simulink model "pry_grasp_source"  (R2018b)
settings: Solver=FixedStepDiscrete  StartTime=0.0  StopTime=Inf  FixedStep=0.001  RelTol=1e-3
PostLoadFcn:
  | , if any(exist('dsrtsu_mdlpostloadfcn', 'file') ~= 0), dsrtsu_mdlpostloadfcn('Execute', bdroot); end,
undefined symbols (not defined in the file): b, Coulomb_friction, parallel_grasp, q1ini, q2ini, theta1, theta2, theta5, theta6, viscous_friction
libraries: simulink x26
(part 3 of 3)

== system pry_grasp_source/phase700/Enabled Subsystem7/Subsystem ==
  note: 关节6弹簧特性
  note: 关节5弹簧特性
  initial_angle : Inport
  end_angle : Inport  Port=2
  end_time : Inport  Port=3
  time : Inport  Port=4
  angular_vel : Inport  Port=5
  current_angle : Inport  Port=6
  Enable : EnablePort
  Demux : Demux  Outputs=8
  Demux1 : Demux  Outputs=8
  MATLAB Function : MATLAB Function  TreatAsAtomicUnit=on
  Mux : Mux  Inputs=8
  P5 : Subsystem
  P6 : Subsystem
  PID1 : Subsystem
  PID2 : Subsystem
  PID3 : Subsystem
  PID4 : Subsystem
  PID7 : Subsystem
  PID8 : Subsystem
  Sum2 : Sum  Inputs=|+-
  angle2 down1 : Constant  Value=2
  angle2 down2 : Constant  Value=2
  torque_out : Outport  OutputWhenDisabled=reset  InitialOutput=[0 0 0 0 0 0 0 0]
  wires:
  initial_angle/1 -> MATLAB Function/1(initial_q)
  end_angle/1 -> MATLAB Function/2(end_q)
  time/1 -> MATLAB Function/4(time)
  end_time/1 -> MATLAB Function/3(end_time)
  angular_vel/1 -> Demux1/1
  MATLAB Function/1(angle_ref_out) -> Sum2/1
  Sum2/1 -> Demux/1
  current_angle/1 -> Sum2/2
  Mux/1 -> torque_out/1
  Demux/1 -> PID1/1(angle_error)
  Demux1/1 -> PID1/2(angular_vel)
  PID1/1(torque) -> Mux/1
  Demux/3 -> PID3/1(angle_error)
  Demux/4 -> PID4/1(angle_error)
  PID3/1(torque) -> Mux/3
  PID4/1(torque) -> Mux/4
  Demux1/3 -> PID3/2(angular_vel)
  Demux1/4 -> PID4/2(angular_vel)
  Demux/7 -> PID7/1(angle_error)
  Demux/8 -> PID8/1(angle_error)
  PID7/1(torque) -> Mux/7
  PID8/1(torque) -> Mux/8
  Demux1/7 -> PID7/2(angular_vel)
  Demux1/8 -> PID8/2(angular_vel)
  PID2/1(torque) -> Mux/2
  angle2 down1/1 -> P6/1(angle_error)
  P6/1(torque6) -> Mux/6
  P5/1(torque6) -> Mux/5
  Demux/2 -> PID2/1(angle_error)
  Demux1/2 -> PID2/2(angular_vel)
  angle2 down2/1 -> P5/1(angle_error)

== system pry_grasp_source/phase700/Enabled Subsystem7/Triggered Subsystem ==
  angle_In1 : Inport
  angle_ref_In2 : Inport  Port=2
  end_time_In3 : Inport  Port=3
  Trigger : TriggerPort  VariantControl=Variant
  angle_Out1 : Outport  InitialOutput=0
  angle_ref_Out2 : Outport  Port=2  InitialOutput=0
  end_time_Out3 : Outport  Port=3  InitialOutput=0
  wires:
  angle_In1/1 -> angle_Out1/1
  angle_ref_In2/1 -> angle_ref_Out2/1
  end_time_In3/1 -> end_time_Out3/1

== system pry_grasp_source/phase700/Subsystem1/Triggered Subsystem3 ==
  Trigger : TriggerPort  VariantControl=(inherit)
  Constant : Constant  Value=[0 1]
  Data Store Read : DataStoreRead  Priority=3  DataStoreName=phase_num
  Data Store Write : DataStoreWrite  DataStoreName=phase_num
  Sum : Sum  Inputs=|++
  wires:
  Data Store Read/1 -> Sum/1
  Sum/1 -> Data Store Write/1
  Constant/1 -> Sum/2

== system pry_grasp_source/phase90/Enabled Subsystem4/Subsystem1 ==
  note: 使关节5平滑转到相应角度
  note: 使关节2维持相应角度
  note: 关节6弹簧特性
  note: 关节2维持角度
  initial_angle5 : Inport
  end_angle5 : Inport  Port=2
  end_time : Inport  Port=3
  time : Inport  Port=4
  angular5_vel : Inport  Port=5
  current_angle5 : Inport  Port=6
  "angle2 " : Inport  Port=7
  angle1 : Inport  Port=8
  Enable : EnablePort
  Fx_1 : Constant
  Fy_1 : Constant  Value=0.1
  MATLAB Function : MATLAB Function  TreatAsAtomicUnit=on
  MATLAB Function1 : MATLAB Function  TreatAsAtomicUnit=on
  Mux : Mux  Inputs=8
  P6 : Subsystem
  PID5 : Subsystem
  Sum2 : Sum  Inputs=|+-
  angle6 down : Constant  Value=-2
  other tau : Constant  Value=0
  phi_value : Constant  Value=16
  torque : Outport
  wires:
  end_time/1 -> MATLAB Function/3(end_time)
  Sum2/1 -> PID5/1(angle_error)
  initial_angle5/1 -> MATLAB Function/1(initial_q)
  time/1 -> MATLAB Function/4(time)
  current_angle5/1 -> Sum2/2
  angular5_vel/1 -> PID5/2(angular_vel)
  MATLAB Function/1(angle_ref_out) -> Sum2/1
  end_angle5/1 -> MATLAB Function/2(end_q)
  angle6 down/1 -> P6/1(angle_error)
  phi_value/1 -> MATLAB Function1/1(phi_value)
  Mux/1 -> torque/1
  other tau/1 -> Mux/8, Mux/7, Mux/4, Mux/3
  PID5/1(torque) -> Mux/5
  P6/1(torque1) -> Mux/6
  Fx_1/1 -> MATLAB Function1/2(Fx_1)
  Fy_1/1 -> MATLAB Function1/3(Fy_1)
  "angle2 "/1 -> MATLAB Function1/5(theta2_value)
  angle1/1 -> MATLAB Function1/4(theta1_value)
  MATLAB Function1/1(tau1) -> Mux/1
  MATLAB Function1/2(tau2) -> Mux/2

== system pry_grasp_source/phase90/Enabled Subsystem4/Triggered Subsystem ==
  angle5_In : Inport
  angle5_ref : Inport  Port=2
  end_time : Inport  Port=3
  Trigger : TriggerPort  VariantControl=Variant
  angle5_Out : Outport  InitialOutput=0
  angle5_ref_Out : Outport  Port=2  InitialOutput=0
  end_time_Out : Outport  Port=3  InitialOutput=0
  wires:
  angle5_In/1 -> angle5_Out/1
  angle5_ref/1 -> angle5_ref_Out/1
  end_time/1 -> end_time_Out/1

== system pry_grasp_source/prying motion/Enabled Subsystem4/Subsystem1 ==
  pry force : Inport
  "angle2 " : Inport  Port=2
  angle1 : Inport  Port=3
  angle6 : Inport  Port=4
  angle5 : Inport  Port=5
  Enable : EnablePort
  Fy_1_finger1 : Constant  Value=0.1
  Fy_1_finger2 : Constant  Value=0.1
  MATLAB Function1 : MATLAB Function  TreatAsAtomicUnit=on
  MATLAB Function2 : MATLAB Function  TreatAsAtomicUnit=on
  Mux : Mux
  offset : Gain  Gain=0.3
  torque : Outport
  wires:
  Mux/1 -> torque/1
  MATLAB Function1/2(tau2) -> Mux/2
  angle1/1 -> MATLAB Function1/3(theta1_value)
  MATLAB Function1/1(tau1) -> Mux/1
  Fy_1_finger1/1 -> MATLAB Function1/2(Fy_1)
  "angle2 "/1 -> MATLAB Function1/4(theta2_value)
  pry force/1 -> offset/1, MATLAB Function1/1(Fx_1)
  angle6/1 -> MATLAB Function2/4(theta6)
  Fy_1_finger2/1 -> MATLAB Function2/2(Fy_1)
  angle5/1 -> MATLAB Function2/3(theta5)
  offset/1 -> MATLAB Function2/1(Fx_1)
  MATLAB Function2/1(tau5) -> Mux/3
  MATLAB Function2/2(tau6) -> Mux/4

== system pry_grasp_source/pusher drops to detect the table surface/friction_compensation model/PID1 ==
  angle_error : Inport
  angular_vel : Inport  Port=2
  Data Store Read : DataStoreRead  DataStoreName=gain1
  Kd : Gain  Gain=0.0005
  Kp : Gain  Gain=0.15
  Product : Product
  Sum1 : Sum  Inputs=|+-
  torque : Outport
  wires:
  Kd/1 -> Sum1/2
  Sum1/1 -> Product/1
  Product/1 -> torque/1
  Kp/1 -> Sum1/1
  angle_error/1 -> Kp/1
  angular_vel/1 -> Kd/1
  Data Store Read/1 -> Product/2

== system pry_grasp_source/pusher drops to detect the table surface/friction_compensation model/PID2 ==
  angle_error : Inport
  angular_vel : Inport  Port=2
  Data Store Read : DataStoreRead  DataStoreName=gain2
  Kd : Gain  Gain=0.0005
  Kp : Gain  Gain=0.15
  Product : Product
  Sum1 : Sum  Inputs=|+-
  torque : Outport
  wires:
  Kd/1 -> Sum1/2
  Sum1/1 -> Product/1
  Product/1 -> torque/1
  Kp/1 -> Sum1/1
  angle_error/1 -> Kp/1
  angular_vel/1 -> Kd/1
  Data Store Read/1 -> Product/2

== system pry_grasp_source/pusher drops to detect the table surface/friction_compensation model/PID6 ==
  angle_error : Inport
  angular_vel : Inport  Port=2
  Data Store Read : DataStoreRead  DataStoreName=gain6
  Kd : Gain  Gain=0.0005
  Kp : Gain  Gain=0.15
  Product : Product
  Sum1 : Sum  Inputs=|+-
  torque : Outport
  wires:
  Kd/1 -> Sum1/2
  Sum1/1 -> Product/1
  Product/1 -> torque/1
  Kp/1 -> Sum1/1
  angle_error/1 -> Kp/1
  angular_vel/1 -> Kd/1
  Data Store Read/1 -> Product/2

== system pry_grasp_source/pusher drops to detect the table surface/friction_compensation model/joint5 torque compensation1 ==
  angular_velocity : Inport
  C5 : Constant  Value=Coulomb_friction  SampleTime=-1
  D5 : Constant  Value=viscous_friction  SampleTime=-1
  Stribeck_friction_model : MATLAB Function  TreatAsAtomicUnit=on
  torque_out : Outport  OutputWhenDisabled=reset  InitialOutput=0
  wires:
  angular_velocity/1 -> Stribeck_friction_model/3(angular_vel)
  C5/1 -> Stribeck_friction_model/1(C)
  D5/1 -> Stribeck_friction_model/2(D)
  Stribeck_friction_model/1(torque_out) -> torque_out/1

== system pry_grasp_source/pusher pushes object/Subsystem1/Triggered Subsystem3 ==
  Trigger : TriggerPort  VariantControl=(inherit)
  Constant : Constant  Value=[0 1]
  Data Store Read : DataStoreRead  Priority=3  DataStoreName=phase_num
  Data Store Write : DataStoreWrite  DataStoreName=phase_num
  Sum : Sum  Inputs=|++
  wires:
  Data Store Read/1 -> Sum/1
  Sum/1 -> Data Store Write/1
  Constant/1 -> Sum/2

== system pry_grasp_source/return to initial angle/Enabled Subsystem7/Subsystem ==
  initial_angle : Inport
  end_angle : Inport  Port=2
  end_time : Inport  Port=3
  time : Inport  Port=4
  angular_vel : Inport  Port=5
  current_angle : Inport  Port=6
  Enable : EnablePort
  Demux : Demux  Outputs=1
  Demux1 : Demux  Outputs=1
  MATLAB Function : MATLAB Function  TreatAsAtomicUnit=on
  Mux : Mux
  PID2 : Subsystem
  Sum2 : Sum  Inputs=|+-
  torque_out : Outport  OutputWhenDisabled=reset  InitialOutput=[0 0 0 0 0 0 0 0]
  wires:
  initial_angle/1 -> MATLAB Function/1(initial_q)
  end_angle/1 -> MATLAB Function/2(end_q)
  time/1 -> MATLAB Function/4(time)
  end_time/1 -> MATLAB Function/3(end_time)
  angular_vel/1 -> Demux1/1
  MATLAB Function/1(angle_ref_out) -> Sum2/1
  Sum2/1 -> Demux/1
  current_angle/1 -> Sum2/2
  Mux/1 -> torque_out/1
  Demux/1 -> PID2/1(angle_error)
  PID2/1(torque) -> Mux/2
  Demux1/1 -> PID2/2(angular_vel)

== system pry_grasp_source/return to initial angle/Enabled Subsystem7/Triggered Subsystem ==
  angle_In1 : Inport
  angle_ref_In2 : Inport  Port=2
  end_time_In3 : Inport  Port=3
  Trigger : TriggerPort  VariantControl=Variant
  angle_Out1 : Outport  InitialOutput=0
  angle_ref_Out2 : Outport  Port=2  InitialOutput=0
  end_time_Out3 : Outport  Port=3  InitialOutput=0
  wires:
  angle_In1/1 -> angle_Out1/1
  angle_ref_In2/1 -> angle_ref_Out2/1
  end_time_In3/1 -> end_time_Out3/1

== system pry_grasp_source/return to initial position/Enabled Subsystem7/Subsystem ==
  initial_angle : Inport
  end_angle : Inport  Port=2
  end_time : Inport  Port=3
  time : Inport  Port=4
  angular_vel : Inport  Port=5
  current_angle : Inport  Port=6
  Enable : EnablePort
  Demux : Demux  Outputs=1
  MATLAB Function : MATLAB Function  TreatAsAtomicUnit=on
  Mux : Mux
  PID1 : Subsystem
  Sum2 : Sum  Inputs=|+-
  tau1 : Gain
  tau_out : Outport
  wires:
  initial_angle/1 -> MATLAB Function/1(initial_q)
  end_angle/1 -> MATLAB Function/2(end_q)
  time/1 -> MATLAB Function/4(time)
  end_time/1 -> MATLAB Function/3(end_time)
  MATLAB Function/1(angle_ref_out) -> Sum2/1
  Sum2/1 -> Demux/1
  current_angle/1 -> Sum2/2
  Mux/1 -> tau_out/1
  Demux/1 -> PID1/1(angle_error)
  angular_vel/1 -> PID1/2(angular_vel)
  PID1/1(torque) -> tau1/1, Mux/1

== system pry_grasp_source/return to initial position/Enabled Subsystem7/Triggered Subsystem ==
  angle_In1 : Inport
  angle_ref_In2 : Inport  Port=2
  end_time_In3 : Inport  Port=3
  Trigger : TriggerPort  VariantControl=Variant
  angle_Out1 : Outport  InitialOutput=0
  angle_ref_Out2 : Outport  Port=2  InitialOutput=0
  end_time_Out3 : Outport  Port=3  InitialOutput=0
  wires:
  angle_In1/1 -> angle_Out1/1
  angle_ref_In2/1 -> angle_ref_Out2/1
  end_time_In3/1 -> end_time_Out3/1

== system pry_grasp_source/tentatively push/Enabled Subsystem1/Subsystem1 ==
  note: 使关节5平滑转到相应角度
  note: desired y
  initial angle : Inport
  end_angle : Inport  Port=2
  end_time : Inport  Port=3
  time : Inport  Port=4
  current angle : Inport  Port=5
  angular_vel : Inport  Port=6
  phase time : Inport  Port=7
  Enable : EnablePort
  Constant2 : Constant  Value=0
  Demux : Demux  Outputs=8
  Demux1 : Demux  Outputs=2
  Gain : Gain  Gain=b
  MATLAB Function : MATLAB Function  TreatAsAtomicUnit=on
  MATLAB Function3 : MATLAB Function  TreatAsAtomicUnit=on
  MATLAB Function4 : MATLAB Function  TreatAsAtomicUnit=on
  Mux : Mux
  Mux{1..4} (4 alike) : Mux  Inputs=2
  PID1 : Subsystem
  PID2 : Subsystem
  Sum : Sum  Inputs=|+-
  Sum1 : Sum  Inputs=|+-
  Sum2 : Sum  Inputs=|+-
  Sum3 : Sum  Inputs=|++
  Sum4 : Sum  Inputs=|++
  measured Fx : Constant  Value=0
  measured Fy : Constant  Value=0.1
  torque : Outport
  wires:
  end_time/1 -> MATLAB Function/3(end_time)
  initial angle/1 -> MATLAB Function/1(initial_q)
  time/1 -> MATLAB Function/4(time)
  current angle/1 -> Sum2/2
  MATLAB Function/1(angle_ref_out) -> Sum2/1
  end_angle/1 -> MATLAB Function/2(end_q)
  Mux/1 -> torque/1
  PID1/1(torque) -> Mux/1
  PID2/1(torque) -> Mux/2
  Sum2/1 -> Demux/1
  Demux/1 -> PID1/1(angle_error)
  Demux/2 -> PID2/1(angle_error)
  angular_vel/1 -> Demux1/1
  Demux1/1 -> PID1/2(angular_vel)
  Demux1/2 -> PID2/2(angular_vel)
  Mux1/1 -> Sum/1
  measured Fy/1 -> Mux2/2
  Mux2/1 -> Sum/2
  MATLAB Function3/2(tau6f) -> Sum4/2
  MATLAB Function4/1(tau5s) -> Sum3/1
  Mux3/1 -> Sum1/1
  Sum/1 -> MATLAB Function3/1(F_e)
  measured Fx/1 -> Mux2/1
  [P_x] -> Mux4/1
  Sum1/1 -> MATLAB Function4/1(P_e)
  [P_y] -> Mux4/2
  Gain/1 -> Mux3/1
  MATLAB Function3/1(tau5f) -> Sum3/2
  Constant2/1 -> Mux3/2
  MATLAB Function4/2(tau6s) -> Sum4/1
  [F_yd] -> Mux1/2
  phase time/1 -> Gain/1
  Sum4/1 -> Mux/4
  [F_xd] -> Mux1/1
  Mux4/1 -> Sum1/2
  Sum3/1 -> Mux/3

== system pry_grasp_source/tentatively push/Enabled Subsystem1/Triggered Subsystem ==
  angle_In : Inport
  angle_ref : Inport  Port=2
  end_time : Inport  Port=3
  Trigger : TriggerPort  VariantControl=Variant
  angle_Out : Outport  InitialOutput=0
  angle_ref_Out : Outport  Port=2  InitialOutput=0
  end_time_Out : Outport  Port=3  InitialOutput=0
  wires:
  angle_In/1 -> angle_Out/1
  angle_ref/1 -> angle_ref_Out/1
  end_time/1 -> end_time_Out/1

== system pry_grasp_source/phase1/Enabled Subsystem7/Subsystem/PID1 ==
  angle_error : Inport
  angular_vel : Inport  Port=2
  Data Store Read : DataStoreRead  DataStoreName=gain1
  Kd : Gain  Gain=0.0005
  Kp : Gain  Gain=0.15
  Product : Product
  Sum1 : Sum  Inputs=|+-
  torque : Outport
  wires:
  Kd/1 -> Sum1/2
  Sum1/1 -> Product/1
  Product/1 -> torque/1
  Kp/1 -> Sum1/1
  angle_error/1 -> Kp/1
  angular_vel/1 -> Kd/1
  Data Store Read/1 -> Product/2

== system pry_grasp_source/phase1/Enabled Subsystem7/Subsystem/PID2 ==
  angle_error : Inport
  angular_vel : Inport  Port=2
  Data Store Read : DataStoreRead  DataStoreName=gain2
  Kd2 : Gain  Gain=0.0002
  Kp2 : Gain  Gain=0.08
  Product : Product
  Sum1 : Sum  Inputs=|+-
  torque : Outport
  wires:
  Kp2/1 -> Sum1/1
  angular_vel/1 -> Kd2/1
  Product/1 -> torque/1
  Kd2/1 -> Sum1/2
  angle_error/1 -> Kp2/1
  Data Store Read/1 -> Product/2
  Sum1/1 -> Product/1

== system pry_grasp_source/phase1/Enabled Subsystem7/Subsystem/PID3 ==
  angle_error : Inport
  angular_vel : Inport  Port=2
  Kd : Gain  Gain=0.0005
  Kp : Gain  Gain=0.15
  Sum1 : Sum  Inputs=|+-
  gain : Gain  Gain=0.5
  torque : Outport
  wires:
  Kd/1 -> Sum1/2
  Sum1/1 -> gain/1
  gain/1 -> torque/1
  Kp/1 -> Sum1/1
  angle_error/1 -> Kp/1
  angular_vel/1 -> Kd/1

== system pry_grasp_source/phase1/Enabled Subsystem7/Subsystem/PID4 ==
  angle_error : Inport
  angular_vel : Inport  Port=2
  Kd2 : Gain  Gain=0.0002
  Kp2 : Gain  Gain=0.08
  Sum1 : Sum  Inputs=|+-
  gain : Gain  Gain=0.5
  torque : Outport
  wires:
  Kp2/1 -> Sum1/1
  angular_vel/1 -> Kd2/1
  Sum1/1 -> gain/1
  gain/1 -> torque/1
  Kd2/1 -> Sum1/2
  angle_error/1 -> Kp2/1

== system pry_grasp_source/phase1/Enabled Subsystem7/Subsystem/PID5 ==
  angle_error : Inport
  angular_vel : Inport  Port=2
  Data Store Read : DataStoreRead  DataStoreName=gain5
  Kd : Gain  Gain=0.0005
  Kp : Gain  Gain=0.15
  Product : Product
  Sum1 : Sum  Inputs=|+-
  torque : Outport
  wires:
  Kd/1 -> Sum1/2
  Kp/1 -> Sum1/1
  angle_error/1 -> Kp/1
  angular_vel/1 -> Kd/1
  Data Store Read/1 -> Product/2
  Sum1/1 -> Product/1
  Product/1 -> torque/1

== system pry_grasp_source/phase1/Enabled Subsystem7/Subsystem/PID6 ==
  angle_error : Inport
  angular_vel : Inport  Port=2
  Data Store Read : DataStoreRead  DataStoreName=gain6
  Kd2 : Gain  Gain=0.0002
  Kp2 : Gain  Gain=0.08
  Product : Product
  Sum1 : Sum  Inputs=|+-
  torque : Outport
  wires:
  Kp2/1 -> Sum1/1
  angular_vel/1 -> Kd2/1
  Sum1/1 -> Product/1
  Product/1 -> torque/1
  Kd2/1 -> Sum1/2
  angle_error/1 -> Kp2/1
  Data Store Read/1 -> Product/2

== system pry_grasp_source/phase1/Enabled Subsystem7/Subsystem/PID7 ==
  angle_error : Inport
  angular_vel : Inport  Port=2
  Kd : Gain  Gain=0.0005
  Kp : Gain  Gain=0.15
  Sum1 : Sum  Inputs=|+-
  gain : Gain  Gain=0.5
  torque : Outport
  wires:
  Kd/1 -> Sum1/2
  Sum1/1 -> gain/1
  gain/1 -> torque/1
  Kp/1 -> Sum1/1
  angle_error/1 -> Kp/1
  angular_vel/1 -> Kd/1

== system pry_grasp_source/phase1/Enabled Subsystem7/Subsystem/PID8 ==
  angle_error : Inport
  angular_vel : Inport  Port=2
  Kd : Gain  Gain=0.0005
  Kp : Gain  Gain=0.15
  Sum1 : Sum  Inputs=|+-
  gain : Gain  Gain=0.5
  torque : Outport
  wires:
  Kd/1 -> Sum1/2
  Sum1/1 -> gain/1
  gain/1 -> torque/1
  Kp/1 -> Sum1/1
  angle_error/1 -> Kp/1
  angular_vel/1 -> Kd/1

== system pry_grasp_source/phase1-1/Enabled Subsystem7/Subsystem/PID1 ==
  angle_error : Inport
  angular_vel : Inport  Port=2
  Data Store Read : DataStoreRead  DataStoreName=gain1
  Kd : Gain  Gain=0.0005
  Kp : Gain  Gain=0.15
  Product : Product
  Sum1 : Sum  Inputs=|+-
  torque : Outport
  wires:
  Kd/1 -> Sum1/2
  Sum1/1 -> Product/1
  Product/1 -> torque/1
  Kp/1 -> Sum1/1
  angle_error/1 -> Kp/1
  angular_vel/1 -> Kd/1
  Data Store Read/1 -> Product/2

== system pry_grasp_source/phase1-1/Enabled Subsystem7/Subsystem/PID2 ==
  angle_error : Inport
  angular_vel : Inport  Port=2
  Data Store Read : DataStoreRead  DataStoreName=gain2
  Kd2 : Gain  Gain=0.0002
  Kp2 : Gain  Gain=0.08
  Product : Product
  Sum1 : Sum  Inputs=|+-
  torque : Outport
  wires:
  Kp2/1 -> Sum1/1
  angular_vel/1 -> Kd2/1
  Product/1 -> torque/1
  Kd2/1 -> Sum1/2
  angle_error/1 -> Kp2/1
  Data Store Read/1 -> Product/2
  Sum1/1 -> Product/1

== system pry_grasp_source/phase1-1/Enabled Subsystem7/Subsystem/PID3 ==
  angle_error : Inport
  angular_vel : Inport  Port=2
  Kd : Gain  Gain=0.0005
  Kp : Gain  Gain=0.15
  Sum1 : Sum  Inputs=|+-
  gain : Gain  Gain=0.5
  torque : Outport
  wires:
  Kd/1 -> Sum1/2
  Sum1/1 -> gain/1
  gain/1 -> torque/1
  Kp/1 -> Sum1/1
  angle_error/1 -> Kp/1
  angular_vel/1 -> Kd/1

== system pry_grasp_source/phase1-1/Enabled Subsystem7/Subsystem/PID4 ==
  angle_error : Inport
  angular_vel : Inport  Port=2
  Kd2 : Gain  Gain=0.0002
  Kp2 : Gain  Gain=0.08
  Sum1 : Sum  Inputs=|+-
  gain : Gain  Gain=0.5
  torque : Outport
  wires:
  Kp2/1 -> Sum1/1
  angular_vel/1 -> Kd2/1
  Sum1/1 -> gain/1
  gain/1 -> torque/1
  Kd2/1 -> Sum1/2
  angle_error/1 -> Kp2/1

== system pry_grasp_source/phase1-1/Enabled Subsystem7/Subsystem/PID5 ==
  angle_error : Inport
  angular_vel : Inport  Port=2
  Data Store Read : DataStoreRead  DataStoreName=gain5
  Kd : Gain  Gain=0.0005
  Kp : Gain  Gain=0.15
  Product : Product
  Sum1 : Sum  Inputs=|+-
  torque : Outport
  wires:
  Kd/1 -> Sum1/2
  Kp/1 -> Sum1/1
  angle_error/1 -> Kp/1
  angular_vel/1 -> Kd/1
  Data Store Read/1 -> Product/2
  Sum1/1 -> Product/1
  Product/1 -> torque/1

== system pry_grasp_source/phase1-1/Enabled Subsystem7/Subsystem/PID6 ==
  angle_error : Inport
  angular_vel : Inport  Port=2
  Data Store Read : DataStoreRead  DataStoreName=gain6
  Kd2 : Gain  Gain=0.0002
  Kp2 : Gain  Gain=0.08
  Product : Product
  Sum1 : Sum  Inputs=|+-
  torque : Outport
  wires:
  Kp2/1 -> Sum1/1
  angular_vel/1 -> Kd2/1
  Sum1/1 -> Product/1
  Product/1 -> torque/1
  Kd2/1 -> Sum1/2
  angle_error/1 -> Kp2/1
  Data Store Read/1 -> Product/2

== system pry_grasp_source/phase1-1/Enabled Subsystem7/Subsystem/PID7 ==
  angle_error : Inport
  angular_vel : Inport  Port=2
  Kd : Gain  Gain=0.0005
  Kp : Gain  Gain=0.15
  Sum1 : Sum  Inputs=|+-
  gain : Gain  Gain=0.5
  torque : Outport
  wires:
  Kd/1 -> Sum1/2
  Sum1/1 -> gain/1
  gain/1 -> torque/1
  Kp/1 -> Sum1/1
  angle_error/1 -> Kp/1
  angular_vel/1 -> Kd/1

== system pry_grasp_source/phase1-1/Enabled Subsystem7/Subsystem/PID8 ==
  angle_error : Inport
  angular_vel : Inport  Port=2
  Kd : Gain  Gain=0.0005
  Kp : Gain  Gain=0.15
  Sum1 : Sum  Inputs=|+-
  gain : Gain  Gain=0.5
  torque : Outport
  wires:
  Kd/1 -> Sum1/2
  Sum1/1 -> gain/1
  gain/1 -> torque/1
  Kp/1 -> Sum1/1
  angle_error/1 -> Kp/1
  angular_vel/1 -> Kd/1

== system pry_grasp_source/phase10/Enabled Subsystem4/Subsystem1/PID1 ==
  angular_vel : Inport
  Kd : Gain  Gain=-0.0005
  Product : Product
  gain_Fx2 : Constant
  torque : Outport
  wires:
  Kd/1 -> Product/1
  Product/1 -> torque/1
  angular_vel/1 -> Kd/1
  gain_Fx2/1 -> Product/2

== system pry_grasp_source/phase10/Enabled Subsystem4/Subsystem1/joint1 friction compensation ==
  angular_velocity : Inport
  C5 : Constant  Value=0.01  SampleTime=-1
  D5 : Constant  Value=0.0007  SampleTime=-1
  Stribeck_friction_model : MATLAB Function  TreatAsAtomicUnit=on
  fric_com_rate : Gain  Gain=0.55
  torque_out : Outport  OutputWhenDisabled=reset  InitialOutput=0
  wires:
  fric_com_rate/1 -> torque_out/1
  Stribeck_friction_model/1(torque_out) -> fric_com_rate/1
  angular_velocity/1 -> Stribeck_friction_model/3(angular_vel)
  C5/1 -> Stribeck_friction_model/1(C)
  D5/1 -> Stribeck_friction_model/2(D)

== system pry_grasp_source/phase10/Enabled Subsystem4/Subsystem1/joint2 torque compensation ==
  angular_velocity : Inport
  C6 : Constant  Value=0.000337  SampleTime=-1
  D6 : Constant  Value=0.0000398  SampleTime=-1
  Stribeck_friction_model : MATLAB Function  TreatAsAtomicUnit=on
  fric_com_rate : Gain  Gain=1.0
  torque_out : Outport  OutputWhenDisabled=reset  InitialOutput=0
  wires:
  fric_com_rate/1 -> torque_out/1
  Stribeck_friction_model/1(torque_out) -> fric_com_rate/1
  angular_velocity/1 -> Stribeck_friction_model/3(angular_vel)
  C6/1 -> Stribeck_friction_model/1(C)
  D6/1 -> Stribeck_friction_model/2(D)

== system pry_grasp_source/phase10/Enabled Subsystem4/Subsystem1/joint5 torque compensation ==
  angular_velocity : Inport
  C5 : Constant  Value=0.012  SampleTime=-1
  D5 : Constant  Value=0.0007  SampleTime=-1
  Stribeck_friction_model : MATLAB Function  TreatAsAtomicUnit=on
  Sum3 : Sum  Inputs=|++
  fric_com_rate : Gain  Gain=1.0
  joint1_tau_offset : Constant  Value=0.0043
  torque_out : Outport  OutputWhenDisabled=reset  InitialOutput=0
  wires:
  Stribeck_friction_model/1(torque_out) -> fric_com_rate/1
  angular_velocity/1 -> Stribeck_friction_model/3(angular_vel)
  C5/1 -> Stribeck_friction_model/1(C)
  D5/1 -> Stribeck_friction_model/2(D)
  joint1_tau_offset/1 -> Sum3/2
  fric_com_rate/1 -> Sum3/1
  Sum3/1 -> torque_out/1

== system pry_grasp_source/phase10/Enabled Subsystem4/Subsystem1/joint6 torque compensation ==
  angular_velocity : Inport
  C6 : Constant  Value=0.000337  SampleTime=-1
  D6 : Constant  Value=0.0000398  SampleTime=-1
  Stribeck_friction_model : MATLAB Function  TreatAsAtomicUnit=on
  fric_com_rate : Gain  Gain=1.0
  torque_out : Outport  OutputWhenDisabled=reset  InitialOutput=0
  wires:
  fric_com_rate/1 -> torque_out/1
  Stribeck_friction_model/1(torque_out) -> fric_com_rate/1
  angular_velocity/1 -> Stribeck_friction_model/3(angular_vel)
  C6/1 -> Stribeck_friction_model/1(C)
  D6/1 -> Stribeck_friction_model/2(D)

== system pry_grasp_source/phase2/Enabled Subsystem7/Subsystem/PID1 ==
  angle_error : Inport
  angular_vel : Inport  Port=2
  Data Store Read : DataStoreRead  DataStoreName=gain1
  Kd : Gain  Gain=0.0005
  Kp : Gain  Gain=0.15
  Product : Product
  Sum1 : Sum  Inputs=|+-
  torque : Outport
  wires:
  Kd/1 -> Sum1/2
  Sum1/1 -> Product/1
  Product/1 -> torque/1
  Kp/1 -> Sum1/1
  angle_error/1 -> Kp/1
  angular_vel/1 -> Kd/1
  Data Store Read/1 -> Product/2

== system pry_grasp_source/phase2/Enabled Subsystem7/Subsystem/PID2 ==
  angle_error : Inport
  angular_vel : Inport  Port=2
  Data Store Read : DataStoreRead  DataStoreName=gain2
  Kd2 : Gain  Gain=0.0002
  Kp2 : Gain  Gain=0.08
  Product : Product
  Sum1 : Sum  Inputs=|+-
  torque : Outport
  wires:
  Kp2/1 -> Sum1/1
  angular_vel/1 -> Kd2/1
  Sum1/1 -> Product/1
  Product/1 -> torque/1
  Kd2/1 -> Sum1/2
  angle_error/1 -> Kp2/1
  Data Store Read/1 -> Product/2

== system pry_grasp_source/phase2/Enabled Subsystem7/Subsystem/PID3 ==
  angle_error : Inport
  angular_vel : Inport  Port=2
  Kd : Gain  Gain=0.0005
  Kp : Gain  Gain=0.15
  Sum1 : Sum  Inputs=|+-
  gain : Gain  Gain=0.5
  torque : Outport
  wires:
  Kd/1 -> Sum1/2
  Sum1/1 -> gain/1
  gain/1 -> torque/1
  Kp/1 -> Sum1/1
  angle_error/1 -> Kp/1
  angular_vel/1 -> Kd/1

== system pry_grasp_source/phase2/Enabled Subsystem7/Subsystem/PID4 ==
  angle_error : Inport
  angular_vel : Inport  Port=2
  Kd2 : Gain  Gain=0.0002
  Kp2 : Gain  Gain=0.08
  Sum1 : Sum  Inputs=|+-
  gain : Gain  Gain=0.5
  torque : Outport
  wires:
  Kp2/1 -> Sum1/1
  angular_vel/1 -> Kd2/1
  Sum1/1 -> gain/1
  gain/1 -> torque/1
  Kd2/1 -> Sum1/2
  angle_error/1 -> Kp2/1

== system pry_grasp_source/phase2/Enabled Subsystem7/Subsystem/PID5 ==
  angle_error : Inport
  angular_vel : Inport  Port=2
  Data Store Read : DataStoreRead  DataStoreName=gain5
  Kd : Gain  Gain=0.0005
  Kp : Gain  Gain=0.15
  Product : Product
  Sum1 : Sum  Inputs=|+-
  torque : Outport
  wires:
  Kd/1 -> Sum1/2
  Sum1/1 -> Product/1
  Product/1 -> torque/1
  Kp/1 -> Sum1/1
  angle_error/1 -> Kp/1
  angular_vel/1 -> Kd/1
  Data Store Read/1 -> Product/2

== system pry_grasp_source/phase2/Enabled Subsystem7/Subsystem/PID6 ==
  angle_error : Inport
  angular_vel : Inport  Port=2
  Data Store Read : DataStoreRead  DataStoreName=gain6
  Kd2 : Gain  Gain=0.0002
  Kp2 : Gain  Gain=0.08
  Product : Product
  Sum1 : Sum  Inputs=|+-
  torque : Outport
  wires:
  Kp2/1 -> Sum1/1
  angular_vel/1 -> Kd2/1
  Sum1/1 -> Product/1
  Product/1 -> torque/1
  Kd2/1 -> Sum1/2
  angle_error/1 -> Kp2/1
  Data Store Read/1 -> Product/2

== system pry_grasp_source/phase2/Enabled Subsystem7/Subsystem/PID7 ==
  angle_error : Inport
  angular_vel : Inport  Port=2
  Kd : Gain  Gain=0.0005
  Kp : Gain  Gain=0.15
  Sum1 : Sum  Inputs=|+-
  gain : Gain  Gain=0.5
  torque : Outport
  wires:
  Kd/1 -> Sum1/2
  Sum1/1 -> gain/1
  gain/1 -> torque/1
  Kp/1 -> Sum1/1
  angle_error/1 -> Kp/1
  angular_vel/1 -> Kd/1

== system pry_grasp_source/phase2/Enabled Subsystem7/Subsystem/PID8 ==
  angle_error : Inport
  angular_vel : Inport  Port=2
  Kd : Gain  Gain=0.0005
  Kp : Gain  Gain=0.15
  Sum1 : Sum  Inputs=|+-
  gain : Gain  Gain=0.5
  torque : Outport
  wires:
  Kd/1 -> Sum1/2
  Sum1/1 -> gain/1
  gain/1 -> torque/1
  Kp/1 -> Sum1/1
  angle_error/1 -> Kp/1
  angular_vel/1 -> Kd/1

== system pry_grasp_source/phase6.1/Enabled Subsystem7/Subsystem/PID1 ==
  angle_error : Inport
  angular_vel : Inport  Port=2
  Data Store Read : DataStoreRead  DataStoreName=gain1
  Kd : Gain  Gain=0.0005
  Kp : Gain  Gain=0.15
  Product : Product
  Sum1 : Sum  Inputs=|+-
  torque : Outport
  wires:
  Kd/1 -> Sum1/2
  Sum1/1 -> Product/1
  Product/1 -> torque/1
  Kp/1 -> Sum1/1
  angle_error/1 -> Kp/1
  angular_vel/1 -> Kd/1
  Data Store Read/1 -> Product/2

== system pry_grasp_source/phase6.1/Enabled Subsystem7/Subsystem/PID2 ==
  angle_error : Inport
  angular_vel : Inport  Port=2
  Data Store Read : DataStoreRead  DataStoreName=gain2
  Kd2 : Gain  Gain=0.0002
  Kp2 : Gain  Gain=0.08
  Product : Product
  Sum1 : Sum  Inputs=|+-
  torque : Outport
  wires:
  Kp2/1 -> Sum1/1
  angular_vel/1 -> Kd2/1
  Product/1 -> torque/1
  Kd2/1 -> Sum1/2
  angle_error/1 -> Kp2/1
  Data Store Read/1 -> Product/2
  Sum1/1 -> Product/1

== system pry_grasp_source/phase6.1/Enabled Subsystem7/Subsystem/PID3 ==
  angle_error : Inport
  angular_vel : Inport  Port=2
  Kd : Gain  Gain=0.0005
  Kp : Gain  Gain=0.15
  Sum1 : Sum  Inputs=|+-
  gain : Gain  Gain=0.5
  torque : Outport
  wires:
  Kd/1 -> Sum1/2
  Sum1/1 -> gain/1
  gain/1 -> torque/1
  Kp/1 -> Sum1/1
  angle_error/1 -> Kp/1
  angular_vel/1 -> Kd/1

== system pry_grasp_source/phase6.1/Enabled Subsystem7/Subsystem/PID4 ==
  angle_error : Inport
  angular_vel : Inport  Port=2
  Kd2 : Gain  Gain=0.0002
  Kp2 : Gain  Gain=0.08
  Sum1 : Sum  Inputs=|+-
  gain : Gain  Gain=0.5
  torque : Outport
  wires:
  Kp2/1 -> Sum1/1
  angular_vel/1 -> Kd2/1
  Sum1/1 -> gain/1
  gain/1 -> torque/1
  Kd2/1 -> Sum1/2
  angle_error/1 -> Kp2/1

== system pry_grasp_source/phase6.1/Enabled Subsystem7/Subsystem/PID5 ==
  angle_error : Inport
  angular_vel : Inport  Port=2
  Data Store Read : DataStoreRead  DataStoreName=gain5
  Kd : Gain  Gain=0.0005
  Kp : Gain  Gain=0.15
  Product : Product
  Sum1 : Sum  Inputs=|+-
  torque : Outport
  wires:
  Kd/1 -> Sum1/2
  Kp/1 -> Sum1/1
  angle_error/1 -> Kp/1
  angular_vel/1 -> Kd/1
  Data Store Read/1 -> Product/2
  Sum1/1 -> Product/1
  Product/1 -> torque/1

== system pry_grasp_source/phase6.1/Enabled Subsystem7/Subsystem/PID6 ==
  angle_error : Inport
  angular_vel : Inport  Port=2
  Data Store Read : DataStoreRead  DataStoreName=gain6
  Kd2 : Gain  Gain=0.0002
  Kp2 : Gain  Gain=0.08
  Product : Product
  Sum1 : Sum  Inputs=|+-
  torque : Outport
  wires:
  Kp2/1 -> Sum1/1
  angular_vel/1 -> Kd2/1
  Sum1/1 -> Product/1
  Product/1 -> torque/1
  Kd2/1 -> Sum1/2
  angle_error/1 -> Kp2/1
  Data Store Read/1 -> Product/2

== system pry_grasp_source/phase6.1/Enabled Subsystem7/Subsystem/PID7 ==
  angle_error : Inport
  angular_vel : Inport  Port=2
  Kd : Gain  Gain=0.0005
  Kp : Gain  Gain=0.15
  Sum1 : Sum  Inputs=|+-
  gain : Gain  Gain=0.5
  torque : Outport
  wires:
  Kd/1 -> Sum1/2
  Sum1/1 -> gain/1
  gain/1 -> torque/1
  Kp/1 -> Sum1/1
  angle_error/1 -> Kp/1
  angular_vel/1 -> Kd/1

== system pry_grasp_source/phase6.1/Enabled Subsystem7/Subsystem/PID8 ==
  angle_error : Inport
  angular_vel : Inport  Port=2
  Kd : Gain  Gain=0.0005
  Kp : Gain  Gain=0.15
  Sum1 : Sum  Inputs=|+-
  gain : Gain  Gain=0.5
  torque : Outport
  wires:
  Kd/1 -> Sum1/2
  Sum1/1 -> gain/1
  gain/1 -> torque/1
  Kp/1 -> Sum1/1
  angle_error/1 -> Kp/1
  angular_vel/1 -> Kd/1

== system pry_grasp_source/phase700/Enabled Subsystem7/Subsystem/P5 ==
  angle_error : Inport
  Data Store Read : DataStoreRead  DataStoreName=gain5
  Kp2 : Gain  Gain=0.08
  Product : Product
  torque6 : Outport
  wires:
  Kp2/1 -> Product/1
  Product/1 -> torque6/1
  angle_error/1 -> Kp2/1
  Data Store Read/1 -> Product/2

== system pry_grasp_source/phase700/Enabled Subsystem7/Subsystem/P6 ==
  angle_error : Inport
  Data Store Read : DataStoreRead  DataStoreName=gain6
  Kp2 : Gain  Gain=0.08
  Product : Product
  torque6 : Outport
  wires:
  Kp2/1 -> Product/1
  Product/1 -> torque6/1
  angle_error/1 -> Kp2/1
  Data Store Read/1 -> Product/2

== system pry_grasp_source/phase700/Enabled Subsystem7/Subsystem/PID1 ==
  angle_error : Inport
  angular_vel : Inport  Port=2
  Data Store Read : DataStoreRead  DataStoreName=gain1
  Kd : Gain  Gain=0.0005
  Kp : Gain  Gain=0.15
  Product : Product
  Sum1 : Sum  Inputs=|+-
  torque : Outport
  wires:
  Kd/1 -> Sum1/2
  Sum1/1 -> Product/1
  Product/1 -> torque/1
  Kp/1 -> Sum1/1
  angle_error/1 -> Kp/1
  angular_vel/1 -> Kd/1
  Data Store Read/1 -> Product/2

== system pry_grasp_source/phase700/Enabled Subsystem7/Subsystem/PID2 ==
  angle_error : Inport
  angular_vel : Inport  Port=2
  Data Store Read : DataStoreRead  DataStoreName=gain2
  Kd : Gain  Gain=0.0005
  Kp : Gain  Gain=0.15
  Product : Product
  Sum1 : Sum  Inputs=|+-
  torque : Outport
  wires:
  Kd/1 -> Sum1/2
  Sum1/1 -> Product/1
  Product/1 -> torque/1
  Kp/1 -> Sum1/1
  angle_error/1 -> Kp/1
  angular_vel/1 -> Kd/1
  Data Store Read/1 -> Product/2

== system pry_grasp_source/phase700/Enabled Subsystem7/Subsystem/PID3 ==
  angle_error : Inport
  angular_vel : Inport  Port=2
  Kd : Gain  Gain=0.0005
  Kp : Gain  Gain=0.15
  Sum1 : Sum  Inputs=|+-
  gain : Gain  Gain=0.5
  torque : Outport
  wires:
  Kd/1 -> Sum1/2
  Sum1/1 -> gain/1
  gain/1 -> torque/1
  Kp/1 -> Sum1/1
  angle_error/1 -> Kp/1
  angular_vel/1 -> Kd/1

== system pry_grasp_source/phase700/Enabled Subsystem7/Subsystem/PID4 ==
  angle_error : Inport
  angular_vel : Inport  Port=2
  Kd2 : Gain  Gain=0.0002
  Kp2 : Gain  Gain=0.08
  Sum1 : Sum  Inputs=|+-
  gain : Gain  Gain=0.5
  torque : Outport
  wires:
  Kp2/1 -> Sum1/1
  angular_vel/1 -> Kd2/1
  Sum1/1 -> gain/1
  gain/1 -> torque/1
  Kd2/1 -> Sum1/2
  angle_error/1 -> Kp2/1

== system pry_grasp_source/phase700/Enabled Subsystem7/Subsystem/PID7 ==
  angle_error : Inport
  angular_vel : Inport  Port=2
  Kd : Gain  Gain=0.0005
  Kp : Gain  Gain=0.15
  Sum1 : Sum  Inputs=|+-
  gain : Gain  Gain=0.5
  torque : Outport
  wires:
  Kd/1 -> Sum1/2
  Sum1/1 -> gain/1
  gain/1 -> torque/1
  Kp/1 -> Sum1/1
  angle_error/1 -> Kp/1
  angular_vel/1 -> Kd/1

== system pry_grasp_source/phase700/Enabled Subsystem7/Subsystem/PID8 ==
  angle_error : Inport
  angular_vel : Inport  Port=2
  Kd : Gain  Gain=0.0005
  Kp : Gain  Gain=0.15
  Sum1 : Sum  Inputs=|+-
  gain : Gain  Gain=0.5
  torque : Outport
  wires:
  Kd/1 -> Sum1/2
  Sum1/1 -> gain/1
  gain/1 -> torque/1
  Kp/1 -> Sum1/1
  angle_error/1 -> Kp/1
  angular_vel/1 -> Kd/1

== system pry_grasp_source/phase90/Enabled Subsystem4/Subsystem1/P6 ==
  angle_error : Inport
  Data Store Read : DataStoreRead  DataStoreName=gain6
  Kp2 : Gain  Gain=0.08
  Product : Product
  torque1 : Outport
  wires:
  Kp2/1 -> Product/1
  Product/1 -> torque1/1
  angle_error/1 -> Kp2/1
  Data Store Read/1 -> Product/2

== system pry_grasp_source/phase90/Enabled Subsystem4/Subsystem1/PID5 ==
  angle_error : Inport
  angular_vel : Inport  Port=2
  Data Store Read : DataStoreRead  DataStoreName=gain5
  Kd5 : Gain  Gain=0.0002
  Kp5 : Gain  Gain=0.08
  Product : Product
  Sum1 : Sum  Inputs=|+-
  torque : Outport
  wires:
  Kp5/1 -> Sum1/1
  angular_vel/1 -> Kd5/1
  Sum1/1 -> Product/1
  Product/1 -> torque/1
  Kd5/1 -> Sum1/2
  angle_error/1 -> Kp5/1
  Data Store Read/1 -> Product/2

== system pry_grasp_source/return to initial angle/Enabled Subsystem7/Subsystem/PID2 ==
  angle_error : Inport
  angular_vel : Inport  Port=2
  Data Store Read : DataStoreRead  DataStoreName=gain2
  Kd2 : Gain  Gain=0.0002
  Kp2 : Gain  Gain=0.08
  Product : Product
  Sum1 : Sum  Inputs=|+-
  torque : Outport
  wires:
  Kp2/1 -> Sum1/1
  angular_vel/1 -> Kd2/1
  Product/1 -> torque/1
  Kd2/1 -> Sum1/2
  angle_error/1 -> Kp2/1
  Data Store Read/1 -> Product/2
  Sum1/1 -> Product/1

== system pry_grasp_source/return to initial position/Enabled Subsystem7/Subsystem/PID1 ==
  angle_error : Inport
  angular_vel : Inport  Port=2
  Data Store Read : DataStoreRead  DataStoreName=gain1
  Kd : Gain  Gain=0.0005
  Kp : Gain  Gain=0.15
  Product : Product
  Sum1 : Sum  Inputs=|+-
  torque : Outport
  wires:
  Kd/1 -> Sum1/2
  Sum1/1 -> Product/1
  Product/1 -> torque/1
  Kp/1 -> Sum1/1
  angle_error/1 -> Kp/1
  angular_vel/1 -> Kd/1
  Data Store Read/1 -> Product/2

== system pry_grasp_source/tentatively push/Enabled Subsystem1/Subsystem1/PID1 ==
  angle_error : Inport
  angular_vel : Inport  Port=2
  Data Store Read : DataStoreRead  DataStoreName=gain1
  Kd5 : Gain  Gain=0.0002
  Kp5 : Gain  Gain=0.08
  Product : Product
  Sum1 : Sum  Inputs=|+-
  torque : Outport
  wires:
  Kp5/1 -> Sum1/1
  angular_vel/1 -> Kd5/1
  Sum1/1 -> Product/1
  Product/1 -> torque/1
  Kd5/1 -> Sum1/2
  angle_error/1 -> Kp5/1
  Data Store Read/1 -> Product/2

== system pry_grasp_source/tentatively push/Enabled Subsystem1/Subsystem1/PID2 ==
  angle_error : Inport
  angular_vel : Inport  Port=2
  Data Store Read : DataStoreRead  DataStoreName=gain2
  Kd5 : Gain  Gain=0.0002
  Kp5 : Gain  Gain=0.08
  Product : Product
  Sum1 : Sum  Inputs=|+-
  torque : Outport
  wires:
  Kp5/1 -> Sum1/1
  angular_vel/1 -> Kd5/1
  Sum1/1 -> Product/1
  Product/1 -> torque/1
  Kd5/1 -> Sum1/2
  angle_error/1 -> Kp5/1
  Data Store Read/1 -> Product/2

== matlab function pry_grasp_source/phase1/Enabled Subsystem7/Subsystem/MATLAB Function ==
  data: initial_q input; angle_ref_out output; end_q input; end_time input; time input
function angle_ref_out = fcn(initial_q, end_q, end_time, time)

tau = time/end_time;

angle_ref_out = initial_q + (end_q-initial_q)*(6*tau^5-15*tau^4+10*tau^3);

== matlab function pry_grasp_source/return to initial position/Enabled Subsystem7/Subsystem/MATLAB Function ==
  data: initial_q input; angle_ref_out output; end_q input; end_time input; time input
function angle_ref_out = fcn(initial_q, end_q, end_time, time)

tau = time/end_time;

angle_ref_out = initial_q + (end_q-initial_q)*(6*tau^5-15*tau^4+10*tau^3);

== matlab function pry_grasp_source/phase10/Enabled Subsystem4/Subsystem1/MATLAB Function3 ==
  data: phi_value input; tau1 output; Fx_1 input; Fy_1 input; theta1_value input; theta2_value input; tau2 output
function [tau1,tau2] = fcn(phi_value, Fx_1, Fy_1, theta1_value,theta2_value)

%Fx_1, Fy_1 代表在surfacce坐标系下的的水平方向与竖直方向的力

l1 = 0.0725;
l2 = 0.06;
phi = phi_value*3.14/180;    %手掌处的旋转角度
theta1 = theta1_value*3.14/180;
theta2 = (theta2_value-90)*3.14/180;
J_R = [cos(phi),sin(phi);-sin(phi),cos(phi)];
F_1 = [Fx_1;Fy_1];
F_0 = J_R*F_1;
J = [-l1*sin(theta1)-l2*sin(theta1+theta2), -l2*sin(theta1+theta2);
    l1*cos(theta1)+l2*cos(theta1+theta2),l2*cos(theta1+theta2)];
J_transpose = transpose(J);
TAU = J_transpose*F_0;
    tau1 = TAU(1,1);
    tau2 = TAU(2,1);

== matlab function pry_grasp_source/phase10/Enabled Subsystem4/Subsystem1/MATLAB Function2 ==
  data: phi_value input; tau5 output; Fx_1 input; Fy_1 input; theta5_value input; theta6_value input; tau6 output
function [tau5,tau6] = fcn(phi_value, Fx_1, Fy_1, theta5_value,theta6_value)

%Fx_1, Fy_1 代表在surfacce坐标系下的的水平方向与竖直方向的力

l1 = 0.0725;
l2 = 0.06;
phi = phi_value*3.14/180;    %手掌处的旋转角度
theta1 = theta5_value*3.14/180;
theta2 = theta6_value*3.14/180;
J_R = [cos(phi),sin(phi);-sin(phi),cos(phi)];
F_1 = [Fx_1;Fy_1];
F_0 = J_R*F_1;
J = [-l1*sin(theta1)-l2*sin(theta1+theta2), -l2*sin(theta1+theta2);
    l1*cos(theta1)+l2*cos(theta1+theta2),l2*cos(theta1+theta2)];
J_transpose = transpose(J);
TAU = J_transpose*F_0;
    tau5 = TAU(1,1);
    tau6 = TAU(2,1);

== matlab function pry_grasp_source/phase700/Enabled Subsystem7/Subsystem/MATLAB Function ==
  data: initial_q input; angle_ref_out output; end_q input; end_time input; time input
function angle_ref_out = fcn(initial_q, end_q, end_time, time)

tau = time/end_time;

angle_ref_out = initial_q + (end_q-initial_q)*(6*tau^5-15*tau^4+10*tau^3);

== matlab function pry_grasp_source/tentatively push/Enabled Subsystem1/Subsystem1/MATLAB Function3 ==
  data: F_e input; tau5f output; tau6f output
function [tau5f,tau6f] = fcn(F_e)

l1 = length1 ;
l2 = length2;

S= [1,0;0,0];
eye = [1,0;0,1];
S_f = eye - S;
Kf = [kf1,0;0,kf2];
J = [-l1*sin(theta1)-l2*sin(theta1+theta2), -l2*sin(theta1+theta2);
    l1*cos(theta1)+l2*cos(theta1+theta2),l2*cos(theta1+theta2)];
tau_f = Kf*transpose(J)*S_f*F_e;


tau5f = tau_f(1,1);
tau6f = tau_f(2,1);

== matlab function pry_grasp_source/phase10/Enabled Subsystem4/Subsystem1/joint5 torque compensation/Stribeck_friction_model ==
  data: C input; D input; angular_vel input; torque_out output
function torque_out = friction_model(C,D,angular_vel)
%#codegen

%vth = 1000;

%if abs(angular_vel)vth
%    Cnl = 3.1*C;
%else
%    Cnl=C;
%end

%%% 速度ベースでクーロン摩擦係数を補正
% 0rad/s:  0.014/C=4.2578
% 23rad/s: C*3.0
% 40rad/s: C*1.5
% 69rad/s: C*1.0
% 97rad/s: C*0.0

%%% 線形近似 %%%

torque_out = ( C ) * sign(angular_vel) + D * angular_vel;

== matlab function pry_grasp_source/phase90/Enabled Subsystem4/Subsystem1/MATLAB Function ==
  data: initial_q input; angle_ref_out output; end_q input; end_time input; time input
function angle_ref_out = fcn(initial_q, end_q, end_time, time)

tau = time/end_time;

angle_ref_out = initial_q + (end_q-initial_q)*(6*tau^5-15*tau^4+10*tau^3);

== matlab function pry_grasp_source/phase90/Enabled Subsystem4/Subsystem1/MATLAB Function1 ==
  data: phi_value input; tau1 output; Fx_1 input; Fy_1 input; theta1_value input; theta2_value input; tau2 output
function [tau1,tau2] = fcn(phi_value, Fx_1, Fy_1, theta1_value,theta2_value)

%Fx_1, Fy_1 代表在surfacce坐标系下的的水平方向与竖直方向的力

l1 = 0.07;
l2 = 0.056;
phi = phi_value*3.14/180;    %手掌处的旋转角度
theta1 = theta1_value*3.14/180;
theta2 = theta2_value*3.14/180;
J_R = [cos(phi),-sin(phi);sin(phi),cos(phi)];
F_1 = [Fx_1;Fy_1];
F_0 = J_R*F_1;
J = [-l1*sin(theta1)-l2*sin(theta1+theta2), -l2*sin(theta1+theta2);
    l1*cos(theta1)+l2*cos(theta1+theta2),l2*cos(theta1+theta2)];
J_transpose = transpose(J);
TAU = J_transpose*F_0;
    tau1 = TAU(1,1);
    tau2 = TAU(2,1);

== matlab function pry_grasp_source/phase10/Enabled Subsystem4/Subsystem1/joint6 torque compensation/Stribeck_friction_model ==
  data: C input; D input; angular_vel input; torque_out output
function torque_out = friction_model(C,D,angular_vel)
%#codegen

%vth = 1000;

%if abs(angular_vel)vth
%    Cnl = 3.1*C;
%else
%    Cnl=C;
%end

%%% 速度ベースでクーロン摩擦係数を補正
% 0rad/s:  0.014/C=4.2578
% 23rad/s: C*3.0
% 40rad/s: C*1.5
% 69rad/s: C*1.0
% 97rad/s: C*0.0

%%% 線形近似 %%%

torque_out =  C  * sign(angular_vel) + D * angular_vel;

== matlab function pry_grasp_source/phase10/Enabled Subsystem4/Subsystem1/joint1 friction compensation/Stribeck_friction_model ==
  data: C input; D input; angular_vel input; torque_out output
function torque_out = friction_model(C,D,angular_vel)
%#codegen

%vth = 1000;

%if abs(angular_vel)vth
%    Cnl = 3.1*C;
%else
%    Cnl=C;
%end

%%% 速度ベースでクーロン摩擦係数を補正
% 0rad/s:  0.014/C=4.2578
% 23rad/s: C*3.0
% 40rad/s: C*1.5
% 69rad/s: C*1.0
% 97rad/s: C*0.0

%%% 線形近似 %%%

torque_out = ( C  ) * sign(angular_vel) + D * angular_vel;

== matlab function pry_grasp_source/phase10/Enabled Subsystem4/Subsystem1/joint2 torque compensation/Stribeck_friction_model ==
  data: C input; D input; angular_vel input; torque_out output
function torque_out = friction_model(C,D,angular_vel)
%#codegen

%vth = 1000;

%if abs(angular_vel)vth
%    Cnl = 3.1*C;
%else
%    Cnl=C;
%end

%%% 速度ベースでクーロン摩擦係数を補正
% 0rad/s:  0.014/C=4.2578
% 23rad/s: C*3.0
% 40rad/s: C*1.5
% 69rad/s: C*1.0
% 97rad/s: C*0.0

%%% 線形近似 %%%

torque_out =  C  * sign(angular_vel) + D * angular_vel;

== matlab function pry_grasp_source/phase11/Enabled Subsystem4/Subsystem1/MATLAB Function1 ==
  data: phi_value input; tau1 output; Fx_1 input; Fy_1 input; theta1_value input; theta2_value input; tau2 output
function [tau1,tau2] = fcn(phi_value, Fx_1, Fy_1, theta1_value,theta2_value)

%Fx_1, Fy_1 代表在surfacce坐标系下的的水平方向与竖直方向的力

l1 = 0.07;
l2 = 0.056;
phi = phi_value*3.14/180;    %手掌处的旋转角度
theta1 = theta1_value*3.14/180;
theta2 = theta2_value*3.14/180;
J_R = [cos(phi),sin(phi);-sin(phi),cos(phi)];
F_1 = [Fx_1;Fy_1];
F_0 = J_R*F_1;
J = [-l1*sin(theta1)-l2*sin(theta1+theta2), -l2*sin(theta1+theta2);
    l1*cos(theta1)+l2*cos(theta1+theta2),l2*cos(theta1+theta2)];
J_transpose = transpose(J);
TAU = J_transpose*F_0;
    tau1 = TAU(1,1);
    tau2 = TAU(2,1);

== matlab function pry_grasp_source/phase11/Enabled Subsystem4/Subsystem1/MATLAB Function2 ==
  data: phi_value input; tau5 output; Fx_1 input; Fy_1 input; theta5_value input; theta6_value input; tau6 output
function [tau5,tau6] = fcn(phi_value, Fx_1, Fy_1, theta5_value,theta6_value)

%Fx_1, Fy_1 代表在surfacce坐标系下的的水平方向与竖直方向的力

l1 = 0.07;
l2 = 0.056;
phi = phi_value*3.14/180;    %手掌处的旋转角度
theta1 = theta5_value*3.14/180;
theta2 = theta6_value*3.14/180;
J_R = [cos(phi),sin(phi);-sin(phi),cos(phi)];
F_1 = [Fx_1;Fy_1];
F_0 = J_R*F_1;
J = [-l1*sin(theta1)-l2*sin(theta1+theta2), -l2*sin(theta1+theta2);
    l1*cos(theta1)+l2*cos(theta1+theta2),l2*cos(theta1+theta2)];
J_transpose = transpose(J);
TAU = J_transpose*F_0;
    tau5 = TAU(1,1);
    tau6 = TAU(2,1);

== matlab function pry_grasp_source/pusher drops to detect the table surface/friction_compensation model/joint5 torque compensation1/Stribeck_friction_model ==
  data: C input; D input; angular_vel input; torque_out output
function torque_out = friction_model(C,D,angular_vel)

torque_out = ( C ) * sign(angular_vel) + D * angular_vel;

== matlab function pry_grasp_source/Hand_counter/MATLAB Function ==
  data: angle1_deg input; delta_x output; angle2_deg input; angle5_deg input; angle6_deg input
function delta_x  = fcn(angle1_deg, angle2_deg, angle5_deg, angle6_deg)


l1 = length1;
l2 = length2;
l3 = length3;
phi = phi_deg*3.14/180;    
J_R = [cos(phi),sin(phi);-sin(phi),cos(phi)];

delta_t = 0.001;    

    theta1_deg = angle1_deg;             %ｽﾇｶﾈ
    theta2_deg = angle2_deg;             %ｽﾇｶﾈ
    theta5_deg = angle5_deg;             %ｽﾇｶﾈ
    theta6_deg = angle6_deg;             %ｽﾇｶﾈ  
    theta1 = theta1_deg*3.14/180;             %ｽﾇｶﾈ
    theta2 = theta2_deg*3.14/180;             %ｽﾇｶﾈ
    theta5 = theta5_deg*3.14/180;             %ｽﾇｶﾈ
    theta6 = theta6_deg*3.14/180;             %ｽﾇｶﾈ
    J = [-l1*sin(theta1)-l2*sin(theta1+theta2), -l2*sin(theta1+theta2);
    l1*cos(theta1)+l2*cos(theta1+theta2),l2*cos(theta1+theta2)];
    J_transpose = transpose(J);
    J_trans_inv = inv(J_transpose);
    gamma = (180-(theta1_deg-phi+theta2_deg))/180*3.14;
    x_1 = -l1*cos(theta1-abs(phi))+l2*cos(gamma);
    x_2 = l3*cos(phi)+l1*cos(theta5+abs(phi))-l2*cos(pi-theta5-theta6-abs(phi));
    delta_x = x_2-x_1;

y = delta_x;

== matlab function pry_grasp_source/return to initial angle/Enabled Subsystem7/Subsystem/MATLAB Function ==
  data: initial_q input; angle_ref_out output; end_q input; end_time input; time input
function angle_ref_out = fcn(initial_q, end_q, end_time, time)

tau = time/end_time;

angle_ref_out = initial_q + (end_q-initial_q)*(6*tau^5-15*tau^4+10*tau^3);

== matlab function pry_grasp_source/phase6.1/Enabled Subsystem7/Subsystem/MATLAB Function ==
  data: initial_q input; angle_ref_out output; end_q input; end_time input; time input
function angle_ref_out = fcn(initial_q, end_q, end_time, time)

tau = time/end_time;

angle_ref_out = initial_q + (end_q-initial_q)*(6*tau^5-15*tau^4+10*tau^3);

== matlab function pry_grasp_source/tentatively push/Enabled Subsystem1/Subsystem1/MATLAB Function ==
  data: initial_q input; angle_ref_out output; end_q input; end_time input; time input
function angle_ref_out = fcn(initial_q, end_q, end_time, time)

tau = time/end_time;

angle_ref_out = initial_q + (end_q-initial_q)*(6*tau^5-15*tau^4+10*tau^3);

== matlab function pry_grasp_source/prying motion/Enabled Subsystem4/Subsystem1/MATLAB Function1 ==
  data: Fx_1 input; tau1 output; Fy_1 input; theta1_value input; theta2_value input; tau2 output
function [tau1,tau2] = fcn( Fx_1, Fy_1, theta1_value,theta2_value)

%Fx_1, Fy_1 代表在surfacce坐标系下的的水平方向与竖直方向的力

l1 = length1 ;
l2 = length2;
theta1 = theta1_value*3.14/180;
theta2 = theta2_value*3.14/180;
J_R = [cos(phi),sin(phi);-sin(phi),cos(phi)];
F_1 = [Fx_1;Fy_1];
F_0 = J_R*F_1;
J = [-l1*sin(theta1)-l2*sin(theta1+theta2), -l2*sin(theta1+theta2);
    l1*cos(theta1)+l2*cos(theta1+theta2),l2*cos(theta1+theta2)];
J_transpose = transpose(J);
TAU = J_transpose*F_0;
    tau1 = TAU(1,1);
    tau2 = TAU(2,1);

== matlab function pry_grasp_source/prying motion/Enabled Subsystem4/Subsystem1/MATLAB Function2 ==
  data: tau5 output; Fx_1 input; Fy_1 input; theta5 input; theta6 input; tau6 output
function [tau5,tau6] = fcn( Fx_1, Fy_1, theta5,theta6)

%Fx_1, Fy_1 代表在surfacce坐标系下的的水平方向与竖直方向的力

l1 = 0.07;
l2 = 0.056;
F_1 = [Fx_1;Fy_1];
J = [-l1*sin(theta5)-l2*sin(theta5+theta6), -l2*sin(theta5+theta6);
    l1*cos(theta5)+l2*cos(theta5+theta6),l2*cos(theta5+theta6)];
J_transpose = transpose(J);
TAU = J_transpose*F_1;
    tau5 = TAU(1,1);
    tau6 = TAU(2,1);

== matlab function pry_grasp_source/prying motion/Enabled Subsystem7/MATLAB Function ==
  data: time input; k input; F_o output; F_end input
function F_o = fcn(time,k,F_end)

F_o = k*time + F_end;

== matlab function pry_grasp_source/tentatively push/Enabled Subsystem1/Subsystem1/MATLAB Function4 ==
  data: P_e input; tau5s output; tau6s output
function [tau5s,tau6s] = fcn(P_e)

l1 = length1 ;
l2 = length2;

S= [1,0;0,0];
Ks = [ks1,0;0,ks2];
J = [-l1*sin(theta1)-l2*sin(theta1+theta2), -l2*sin(theta1+theta2);
    l1*cos(theta1)+l2*cos(theta1+theta2),l2*cos(theta1+theta2)];
tau_p = Ks*transpose(J)*S*P_e;


tau5s = tau_p(1,1);
tau6s = tau_p(2,1);

== matlab function pry_grasp_source/pusher pushes object/Enabled Subsystem4/MATLAB Function1 ==
  data: tau1 output; Fx_1 input; Fy_1 input; theta1_value input; theta2_value input; tau2 output
function [tau1,tau2] = fcn( Fx_1, Fy_1, theta1_value,theta2_value)

%Fx_1, Fy_1 代表在surfacce坐标系下的的水平方向与竖直方向的力

l1 = length1 ;
l2 = length2;
theta1 = theta1_value*3.14/180;
theta2 = theta2_value*3.14/180;
F_1 = [Fx_1;Fy_1];
J = [-l1*sin(theta1)-l2*sin(theta1+theta2), -l2*sin(theta1+theta2);
    l1*cos(theta1)+l2*cos(theta1+theta2),l2*cos(theta1+theta2)];
J_transpose = transpose(J);
TAU = J_transpose*F_0;
    tau1 = TAU(1,1);
    tau2 = TAU(2,1);

== matlab function pry_grasp_source/pusher pushes object/Enabled Subsystem4/MATLAB Function3 ==
  data: F_e input; tau5f output; tau6f output
function [tau5f,tau6f] = fcn(F_e)

l1 = length1 ;
l2 = length2;

S= [1,0;0,0];
eye = [1,0;0,1];
S_f = eye - S;
Kf = [kf1,0;0,kf2];
J = [-l1*sin(theta1)-l2*sin(theta1+theta2), -l2*sin(theta1+theta2);
    l1*cos(theta1)+l2*cos(theta1+theta2),l2*cos(theta1+theta2)];
tau_f = Kf*transpose(J)*S_f*F_e;


tau5f = tau_f(1,1);
tau6f = tau_f(2,1);

== matlab function pry_grasp_source/pusher pushes object/Enabled Subsystem4/MATLAB Function4 ==
  data: P_e input; tau5s output; tau6s output
function [tau5s,tau6s] = fcn(P_e)

l1 = length1 ;
l2 = length2;

S= [1,0;0,0];
Ks = [ks1,0;0,ks2];
J = [-l1*sin(theta1)-l2*sin(theta1+theta2), -l2*sin(theta1+theta2);
    l1*cos(theta1)+l2*cos(theta1+theta2),l2*cos(theta1+theta2)];
tau_p = Ks*transpose(J)*S*P_e;


tau5s = tau_p(1,1);
tau6s = tau_p(2,1);
